simulink model "brain_tumor_controller"  (R2024a)
settings: Solver=VariableStepAuto  StartTime=0.0  StopTime=2.5  RelTol=1e-3
settings Model: Creator=samad  LastModifiedBy=samad

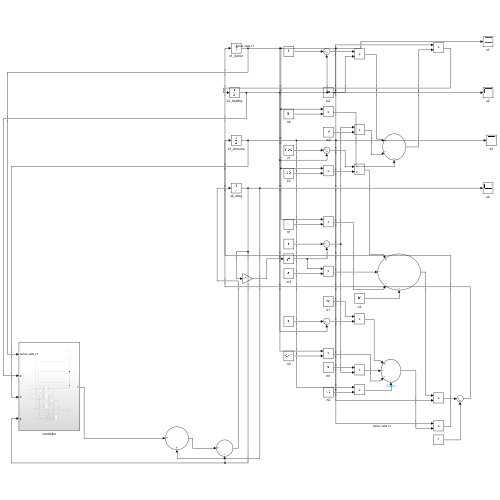
[thumbnail: Simulink's stored preview of the top-level diagram]
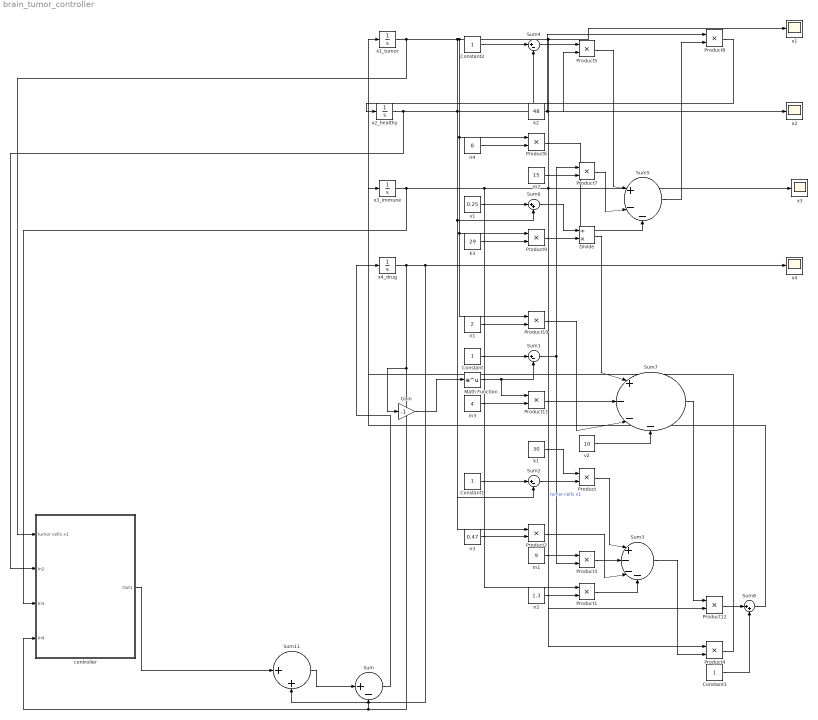
== system brain_tumor_controller ==
  Constant{,1..3} (4 alike) : Constant
  Divide : Product  Inputs=/*
  Gain : Gain  Gain=-1
  Math Function : Math
  Product{,1..12} (13 alike) : Product
  Sum{,1..2,4} (4 alike) : Sum  Inputs=|+-
  Sum11 : Sum  Inputs=|++
  Sum3 : Sum  Inputs=|+---
  Sum5 : Sum  Inputs=|+--
  Sum6 : Sum  Inputs=|++
  Sum7 : Sum  Inputs=|+---
  Sum8 : Sum  Inputs=|++
  controller : Subsystem
  k1 : Constant  Value=30
  k2 : Constant  Value=48
  k3 : Constant  Value=29
  m1 : Constant  Value=9
  m2 : Constant  Value=15
  m3 : Constant  Value=4
  n1 : Constant  Value=2
  n2 : Constant  Value=1.3
  n3 : Constant  Value=0.47
  n4 : Constant  Value=8
  v1 : Constant  Value=0.25
  v2 : Constant  Value=10
  x{1..4} (4 alike) : Scope
  x1_tumor : Integrator  InitialCondition=2.5
  x2_healthy : Integrator  InitialCondition=0.25
  x3_immune : Integrator  InitialCondition=1.55
  x4_drug : Integrator  InitialCondition=2
  wires:
  Sum7/1 -> Product12/1
  m1/1 -> Product3/1
  n3/1 -> Product2/2
  n1/1 -> Product10/2
  n2/1 -> Product1/2
  m2/1 -> Product7/2
  n4/1 -> Product6/2
  k3/1 -> Product9/2
  Divide/1 -> Sum7/1
  Constant/1 -> Sum1/1
  Constant2/1 -> Sum4/1
  Product11/1 -> Sum7/2
  v1/1 -> Sum6/1
  Product1/1 -> Sum3/4
  Product/1 -> Sum3/1
  Product10/1 -> Sum7/3
  m3/1 -> Product11/2
  Math Function/1 -> Sum1/2, Product11/1
  Constant1/1 -> Sum2/1
  Sum3/1 -> Product4/2
  Sum2/1 -> Product/2
  Sum1/1 -> Product3/2, Product7/1
  Sum/1 -> x4_drug/1
  x1_tumor/1 -> controller/1(tumor cells x1), Sum2/2, Sum6/2, Product10/1, Product9/1, Product6/1, Product4/1, x1/1  "tumor cells x1"
  Sum5/1 -> Product8/2
  Sum4/1 -> Product5/1
  Sum6/1 -> Divide/1
  k2/1 -> Product5/2
  Product8/1 -> x2_healthy/1
  Product7/1 -> Sum5/2
  Product9/1 -> Divide/2
  Product6/1 -> Sum5/3
  k1/1 -> Product/1
  Product4/1 -> x1_tumor/1
  Product3/1 -> Sum3/2
  Product5/1 -> Sum5/1
  Product2/1 -> Sum3/3
  v2/1 -> Sum7/4
  Product12/1 -> Sum8/1
  Constant3/1 -> Sum8/2
  Sum8/1 -> x3_immune/1
  Gain/1 -> Math Function/1
  Sum11/1 -> Sum/1
  x4_drug/1 -> controller/4(In4), Sum/2, Gain/1, Sum11/2, x4/1
  x2_healthy/1 -> controller/2(In2), x2/1, Product8/1, Sum4/2, Product2/1
  x3_immune/1 -> controller/3(In3), Product12/2, x3/1, Product1/1
  controller/1(Out1) -> Sum11/1

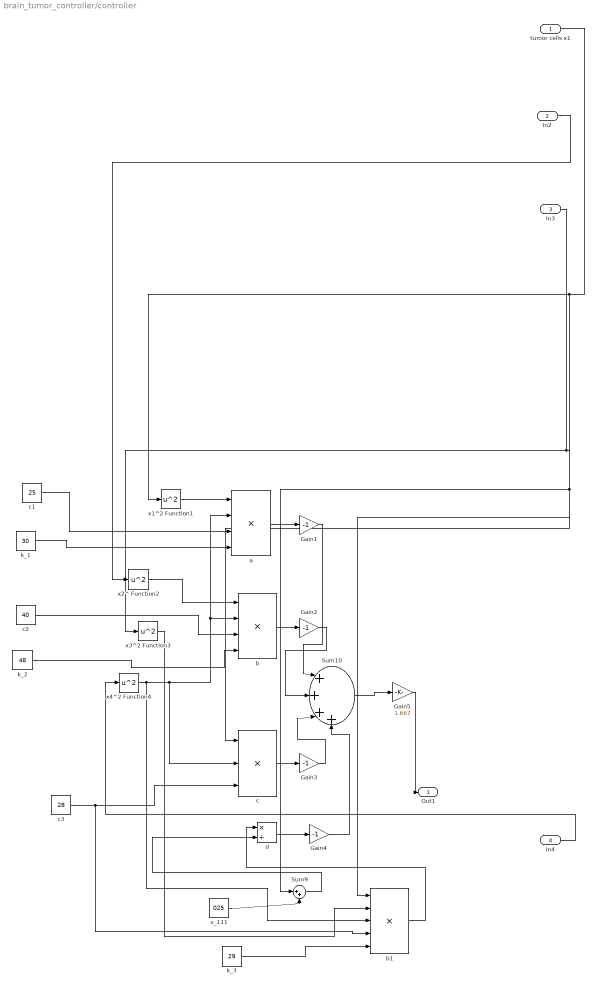
== system brain_tumor_controller/controller ==
  tumor cells x1 : Inport
  In2 : Inport  Port=2
  In3 : Inport  Port=3
  In4 : Inport  Port=4
  Gain{1..4} (4 alike) : Gain  Gain=-1
  Gain5 : Gain  Gain=1.667
  Sum10 : Sum  Inputs=|++++
  Sum9 : Sum  Inputs=|++
  a : Product  Inputs=4
  b : Product  Inputs=4
  b1 : Product  Inputs=5
  c : Product  Inputs=3
  c1 : Constant  Value=25
  c2 : Constant  Value=40
  c3 : Constant  Value=28
  d : Product  Inputs=*/
  k_1 : Constant  Value=30
  k_2 : Constant  Value=48
  k_3 : Constant  Value=29
  v_111 : Constant  Value=025
  x1^2 Function1 : Math  Operator=square
  x2^ Function2 : Math  Operator=square
  x3^2 Function3 : Math  Operator=square
  x4^2 Function4 : Math  Operator=square
  Out1 : Outport
  wires:
  c/1 -> Gain3/1
  x4^2 Function4/1 -> b1/3, c/2, b/2, a/2
  x1^2 Function1/1 -> a/1
  a/1 -> Gain1/1
  b/1 -> Gain2/1
  tumor cells x1/1 -> Sum9/1, b1/1, x1^2 Function1/1
  Gain3/1 -> Sum10/3
  v_111/1 -> Sum9/2
  k_2/1 -> b/4
  k_3/1 -> b1/5
  k_1/1 -> a/4
  b1/1 -> d/1
  Gain1/1 -> Sum10/1
  x3^2 Function3/1 -> b1/2
  c3/1 -> b1/4, c/3
  c2/1 -> b/3
  x2^ Function2/1 -> b/1
  c1/1 -> a/3
  Gain4/1 -> Sum10/4
  d/1 -> Gain4/1
  Gain2/1 -> Sum10/2
  Sum9/1 -> d/2
  In3/1 -> c/1, x3^2 Function3/1
  In4/1 -> x4^2 Function4/1
  Sum10/1 -> Gain5/1
  In2/1 -> x2^ Function2/1
  Gain5/1 -> Out1/1
